simulink model "prob7_214869"  (R2020a)
settings: Solver=VariableStepAuto  StartTime=0.0  StopTime=10.0  RelTol=1e-3
settings Model: Creator=sonal  LastModifiedBy=sonal

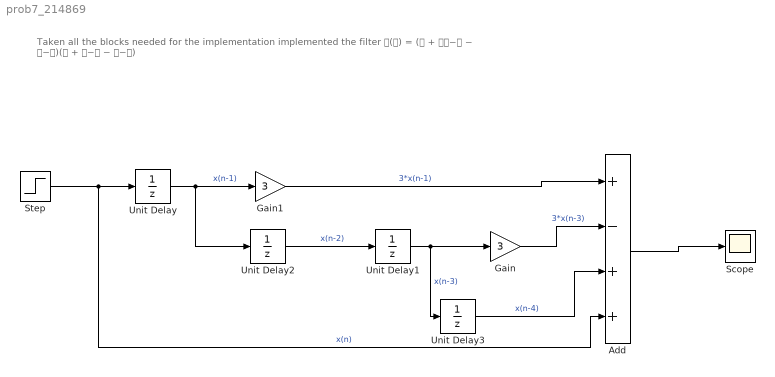
== system prob7_214869 ==
  note: Taken all the blocks needed for the implementation
      | implemented the filter 𝐇(𝐳) = (𝟏 + 𝟐𝐳−𝟏 − 𝐳−𝟐)(𝟏 + 𝐳−𝟏 − 𝐳−𝟐)
  Add : Sum  Inputs=+-++
  Gain : Gain  Gain=3
  Gain1 : Gain  Gain=3
  Scope : Scope
  Step : Step  SampleTime=0
  Unit Delay{,1..3} (4 alike) : UnitDelay  SampleTime=-1  HasFrameUpgradeWarning=on
  wires:
  Step/1 -> Add/4, Unit Delay/1  "x(n)"
  Unit Delay/1 -> Unit Delay2/1, Gain1/1  "x(n-1)"
  Unit Delay2/1 -> Unit Delay1/1  "x(n-2)"
  Unit Delay1/1 -> Unit Delay3/1, Gain/1  "x(n-3)"
  Add/1 -> Scope/1
  Gain1/1 -> Add/1  "3*x(n-1)"
  Gain/1 -> Add/2  "3*x(n-3)"
  Unit Delay3/1 -> Add/3  "x(n-4)"
